simulink model "MARCH_v1"  (R2016a)
settings: Solver=FixedStepDiscrete  StartTime=0.0  StopTime=inf  FixedStep=0.001  RelTol=1e-3
PostLoadFcn:
  | build_location = fullfile(fileparts(which(bdroot)),'build');
  | 
  | set_param(0, 'CacheFolder', build_location);
  | set_param(0, 'CodeGenFolder', build_location);
InitFcn:
  | % Change dir to model location
  | cd(fileparts(which(bdroot)));
  | 
  | % Run init script
  | init_model;
StartFcn:
  | % Make sure we always move back to model folder
  | cd(fileparts(which(bdroot)));
StopFcn:
  | % Make sure we always move back to model folder
  | cd(fileparts(which(bdroot)));
libraries: xpcethercatlib x21
CloseFcn:
  | % Make sure we always move back to model folder
  | cd(fileparts(which(bdroot)));
  | 
  | set_param(0, 'CacheFolder', '');
  | set_param(0, 'CodeGenFolder', '');
PauseFcn:
  | % Make sure we always move back to model folder
  | cd(fileparts(which(bdroot)));
ContinueFcn:
  | % Make sure we always move back to model folder
  | cd(fileparts(which(bdroot)));
settings Model: xpc_rtwmakecfg_data=_xpcethercatlib_  Creator=Projectmarch  LastModifiedBy=Projectmarch
settings SolverCC: EnableConcurrentExecution=on  ConcurrentTasks=on  AutoInsertRateTranBlk=on
settings DataIOCC: LimitDataPoints=on  SaveFinalState=on  SaveFormat=StructureWithTime  InspectSignalLogs=on
settings OptimizationCC: BlockReduction=off  DefaultParameterBehavior=Inlined  OptimizeBlockIOStorage=off  BufferReuse=off  GlobalBufferReuse=off  ExpressionFolding=off  LocalBlockOutputs=off  StateBitsets=on  DataBitsets=on
settings DebuggingCC: AllowSymbolicDim=off
settings HardwareCC: ProdBitPerPointer=32  ProdLargestAtomicFloat=None  ProdWordSize=32  ProdLongLongMode=on  ProdHWDeviceType=Generic->32-bit x86 compatible
settings ModelReferenceCC: PropagateSignalLabelsOutOfModel=off
settings RTWCC: SystemTargetFile=slrt.tlc  TLCOptions=-p0  TemplateMakefile=slrt_default_tmf  Description=Simulink Real-Time  RTWVerbose=off  RTWCompilerOptimization=on
settings SimulinkRealTimeCC: xPCisModelTimeout=off  xPCModelTimeoutSecs=20

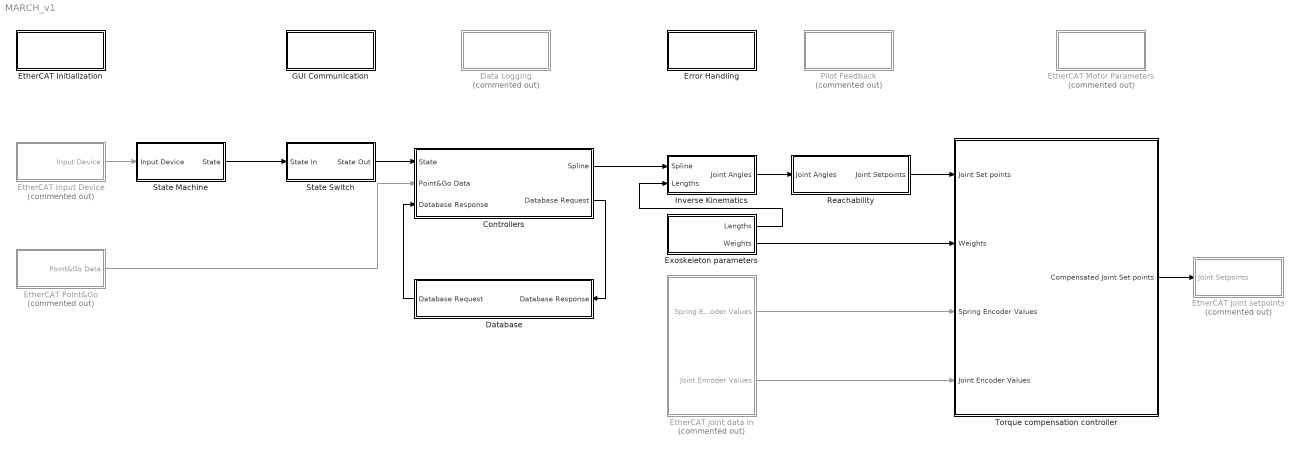
== system MARCH_v1 ==
  Controllers : Subsystem
  Data Logging : Subsystem  Commented=on
  Database : Subsystem
  Error Handling : Subsystem
  EtherCAT Initialization : Subsystem
  EtherCAT Input Device : Subsystem  Commented=on
  EtherCAT Motor Parameters : Subsystem  Commented=on
  EtherCAT Point&Go : Subsystem  Commented=on
  EtherCAT joint data in : Subsystem  Commented=on
  EtherCAT joint setpoints : Subsystem  Commented=on
  Exoskeleton parameters : Subsystem
  GUI Communication : Subsystem
  Inverse Kinematics : Subsystem
  Pilot Feedback : Subsystem  Commented=on
  Reachability : Subsystem
  State Machine : Subsystem
  State Switch : Subsystem
  Torque compensation controller : Subsystem
  wires:
  Torque compensation controller/1(Compensated Joint Set points) -> EtherCAT joint setpoints/1(Joint Setpoints)
  Reachability/1(Joint Setpoints) -> Torque compensation controller/1(Joint Set points)
  Inverse Kinematics/1(Joint Angles) -> Reachability/1(Joint Angles)
  State Switch/1(State Out) -> Controllers/1(State)
  Controllers/1(Spline) -> Inverse Kinematics/1(Spline)
  State Machine/1(State) -> State Switch/1(State In)
  Controllers/2(Database Request) -> Database/1(Database Response)
  Database/1(Database Request) -> Controllers/3(Database Response)
  EtherCAT joint data in/1(Spring Encoder Values) -> Torque compensation controller/3(Spring Encoder Values)
  EtherCAT joint data in/2(Joint Encoder Values) -> Torque compensation controller/4(Joint Encoder Values)
  Exoskeleton parameters/1(Lengths) -> Inverse Kinematics/2(Lengths)
  Exoskeleton parameters/2(Weights) -> Torque compensation controller/2(Weights)
  EtherCAT Input Device/1(Input Device) -> State Machine/1(Input Device)
  EtherCAT Point&Go/1(Point&Go Data) -> Controllers/2(Point&Go Data)

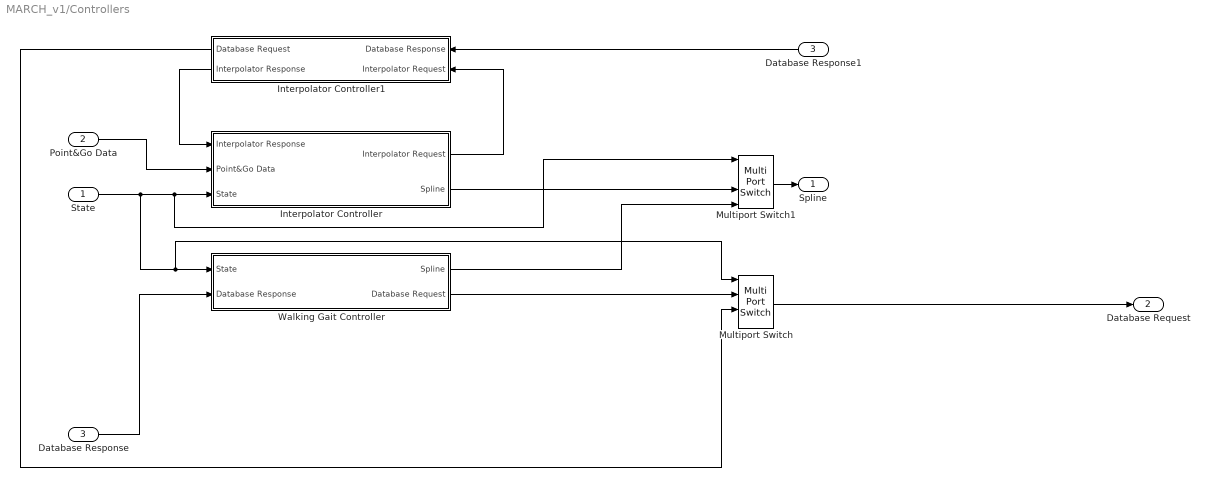
== system MARCH_v1/Controllers ==
  State : Inport
  Point&Go Data : Inport  Port=2
  Database Response : Inport  Port=3
  Database Response1 : InportShadow  Port=3
  Interpolator Controller : Subsystem
  Interpolator Controller1 : Subsystem
  Multiport Switch : MultiPortSwitch
  Multiport Switch1 : MultiPortSwitch
  Walking Gait Controller : Subsystem
  Spline : Outport
  Database Request : Outport  Port=2
  wires:
  State/1 -> Interpolator Controller/3(State), Multiport Switch1/1, Walking Gait Controller/1(State), Multiport Switch/1
  Database Response/1 -> Walking Gait Controller/2(Database Response)
  Walking Gait Controller/1(Spline) -> Multiport Switch1/4
  Interpolator Controller/1(Interpolator Request) -> Interpolator Controller1/2(Interpolator Request)
  Interpolator Controller1/2(Interpolator Response) -> Interpolator Controller/1(Interpolator Response)
  Database Response1/1 -> Interpolator Controller1/1(Database Response)
  Interpolator Controller1/1(Database Request) -> Multiport Switch/3
  Walking Gait Controller/2(Database Request) -> Multiport Switch/2
  Multiport Switch/1 -> Database Request/1
  Interpolator Controller/2(Spline) -> Multiport Switch1/3
  Multiport Switch1/1 -> Spline/1
  Point&Go Data/1 -> Interpolator Controller/2(Point&Go Data)

== system MARCH_v1/Data Logging ==

== system MARCH_v1/Database ==
  Database Response : Inport
  Database Request : Outport

== system MARCH_v1/Error Handling ==

== system MARCH_v1/EtherCAT Initialization ==
  "EtherCAT Init " : xpcethercatlib/EtherCAT Init   Priority=0  config_file=D:\Software\MATLAB\simulink-models\EtherCAT Config files\quad_slave_both_legs_v1.0.xml  device_id=0  pci_bus=0  pci_slot=0  dctuning=0  enaDebug=off  enaDC=on  errLink=off  masterDbg=off  stateChgDbg=off  baseClock=off  masterCfg=off  logFile='c:\dbglog.txt'  sample_time=0.001000

== system MARCH_v1/EtherCAT Input Device ==
  EtherCAT PDO Receive : xpcethercatlib/EtherCAT PDO Receive  Priority=2  sig_name=LHFE.Inputs.jointAngle  sig_offset=208  sig_type=uint32  type_size=32  sig_dim=1  device_id=0  sample_time=0.001000
  Input Device : Outport
  wires:
  EtherCAT PDO Receive/1 -> Input Device/1

== system MARCH_v1/EtherCAT Motor Parameters ==

== system MARCH_v1/EtherCAT Point&Go ==
  EtherCAT PDO Receive : xpcethercatlib/EtherCAT PDO Receive  Priority=2  sig_name=LHFE.Inputs.jointAngle  sig_offset=208  sig_type=uint32  type_size=32  sig_dim=1  device_id=0  sample_time=0.001000
  Point&Go Data : Outport
  wires:
  EtherCAT PDO Receive/1 -> Point&Go Data/1

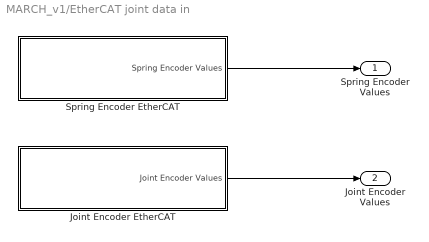
== system MARCH_v1/EtherCAT joint data in ==
  Joint Encoder EtherCAT : Subsystem
  Spring Encoder EtherCAT : Subsystem
  Spring Encoder Values : Outport
  Joint Encoder Values : Outport  Port=2
  wires:
  Spring Encoder EtherCAT/1(Spring Encoder Values) -> Spring Encoder Values/1
  Joint Encoder EtherCAT/1(Joint Encoder Values) -> Joint Encoder Values/1

== system MARCH_v1/EtherCAT joint setpoints ==
  Joint Setpoints : Inport
  EtherCAT Joint Communication : Subsystem
  wires:
  Joint Setpoints/1 -> EtherCAT Joint Communication/1(Joint Setpoints)

== system MARCH_v1/Exoskeleton parameters ==
  Lengths : Outport
  Weights : Outport  Port=2

== system MARCH_v1/GUI Communication ==

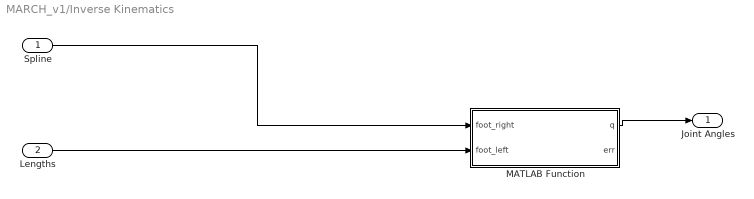
== system MARCH_v1/Inverse Kinematics ==
  Spline : Inport
  Lengths : Inport  Port=2
  MATLAB Function : MATLAB Function  TreatAsAtomicUnit=on
  Joint Angles : Outport
  wires:
  Spline/1 -> MATLAB Function/1(foot_right)
  MATLAB Function/1(q) -> Joint Angles/1
  Lengths/1 -> MATLAB Function/2(foot_left)

== system MARCH_v1/Pilot Feedback ==

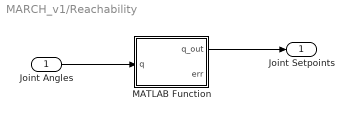
== system MARCH_v1/Reachability ==
  Joint Angles : Inport
  MATLAB Function : MATLAB Function  TreatAsAtomicUnit=on
  Joint Setpoints : Outport
  wires:
  Joint Angles/1 -> MATLAB Function/1(q)
  MATLAB Function/1(q_out) -> Joint Setpoints/1

== system MARCH_v1/State Machine ==
  Input Device : Inport
  Constant : Constant
  State : Outport
  wires:
  Constant/1 -> State/1

== system MARCH_v1/State Switch ==
  State In : Inport
  State Out : Outport
  wires:
  State In/1 -> State Out/1

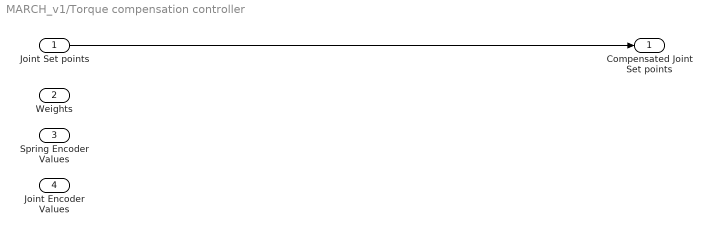
== system MARCH_v1/Torque compensation controller ==
  Joint Set points : Inport
  Weights : Inport  Port=2
  Spring Encoder Values : Inport  Port=3
  Joint Encoder Values : Inport  Port=4
  Compensated Joint Set points : Outport
  wires:
  Joint Set points/1 -> Compensated Joint Set points/1

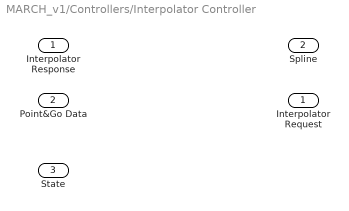
== system MARCH_v1/Controllers/Interpolator Controller ==
  Interpolator Response : Inport
  Point&Go Data : Inport  Port=2
  State : Inport  Port=3
  Interpolator Request : Outport
  Spline : Outport  Port=2

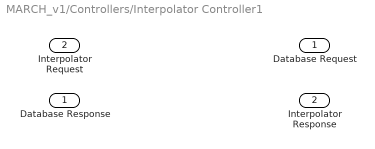
== system MARCH_v1/Controllers/Interpolator Controller1 ==
  Database Response : Inport
  Interpolator Request : Inport  Port=2
  Database Request : Outport
  Interpolator Response : Outport  Port=2

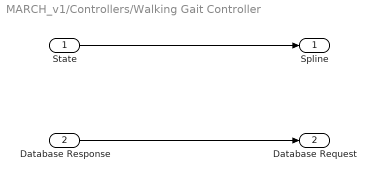
== system MARCH_v1/Controllers/Walking Gait Controller ==
  State : Inport
  Database Response : Inport  Port=2
  Spline : Outport
  Database Request : Outport  Port=2
  wires:
  State/1 -> Spline/1
  Database Response/1 -> Database Request/1

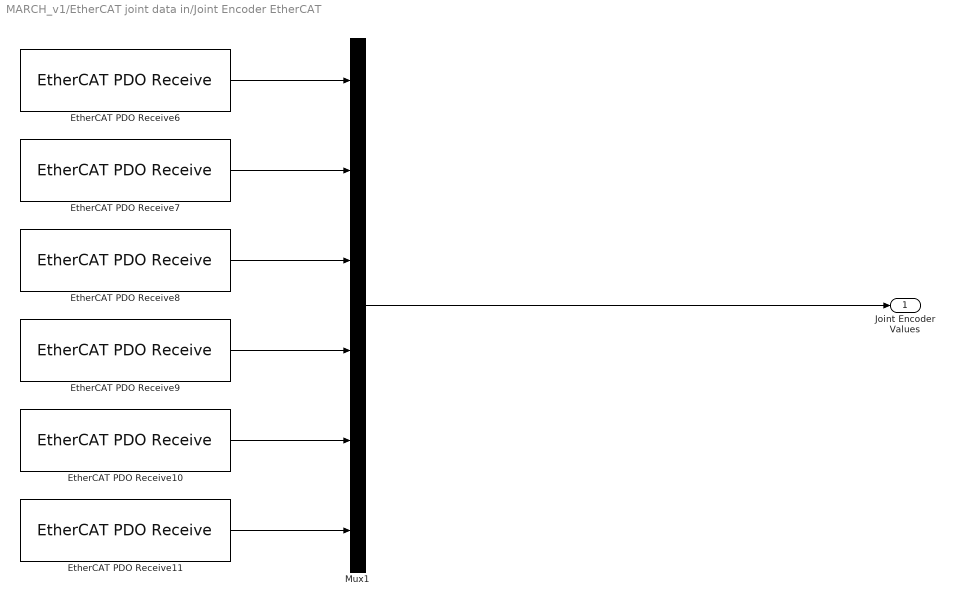
== system MARCH_v1/EtherCAT joint data in/Joint Encoder EtherCAT ==
  EtherCAT PDO Receive{6..11} (6 alike) : xpcethercatlib/EtherCAT PDO Receive  Priority=2  sig_name=Uninitialized Block  sig_offset=144  sig_type=uint8  type_size=8  sig_dim=1  device_id=0  sample_time=0.010000
  Mux1 : Mux  Inputs=6
  Joint Encoder Values : Outport
  wires:
  EtherCAT PDO Receive8/1 -> Mux1/3
  EtherCAT PDO Receive9/1 -> Mux1/4
  EtherCAT PDO Receive7/1 -> Mux1/2
  EtherCAT PDO Receive6/1 -> Mux1/1
  EtherCAT PDO Receive10/1 -> Mux1/5
  EtherCAT PDO Receive11/1 -> Mux1/6
  Mux1/1 -> Joint Encoder Values/1

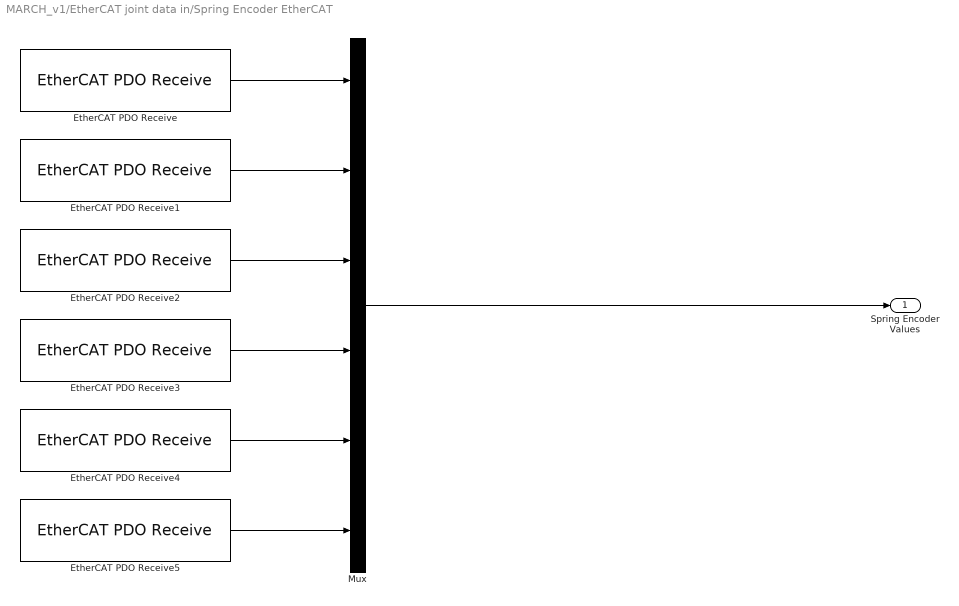
== system MARCH_v1/EtherCAT joint data in/Spring Encoder EtherCAT ==
  EtherCAT PDO Receive{,1..5} (6 alike) : xpcethercatlib/EtherCAT PDO Receive  Priority=2  sig_name=Uninitialized Block  sig_offset=144  sig_type=uint8  type_size=8  sig_dim=1  device_id=0  sample_time=0.010000
  Mux : Mux  Inputs=6
  Spring Encoder Values : Outport
  wires:
  EtherCAT PDO Receive2/1 -> Mux/3
  EtherCAT PDO Receive4/1 -> Mux/5
  Mux/1 -> Spring Encoder Values/1
  EtherCAT PDO Receive5/1 -> Mux/6
  EtherCAT PDO Receive1/1 -> Mux/2
  EtherCAT PDO Receive/1 -> Mux/1
  EtherCAT PDO Receive3/1 -> Mux/4

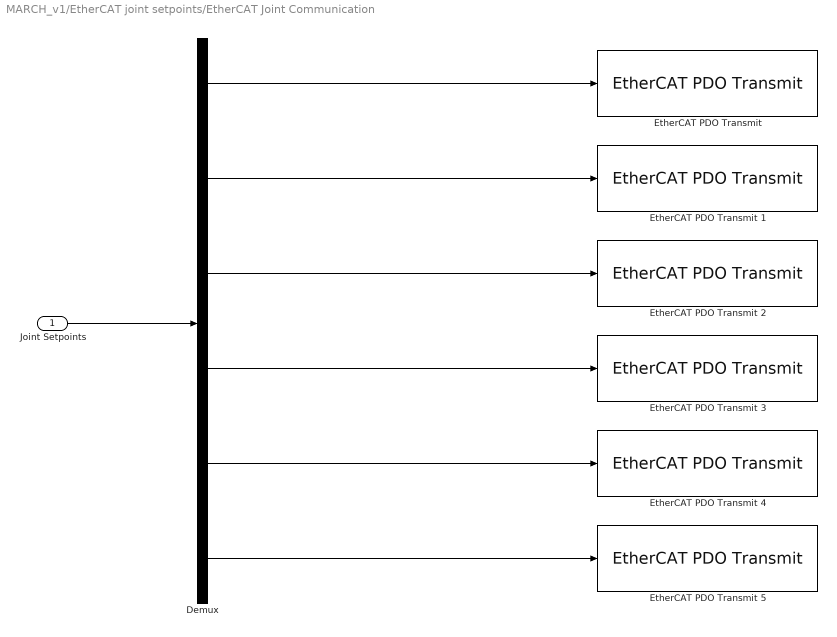
== system MARCH_v1/EtherCAT joint setpoints/EtherCAT Joint Communication ==
  Joint Setpoints : Inport
  Demux : Demux  Outputs=6
  "EtherCAT PDO Transmit " : xpcethercatlib/EtherCAT PDO Transmit   Priority=3  sig_name=LKFE.Outputs.jointSetpoint  sig_offset=496  sig_type=uint32  type_size=32  sig_dim=1  device_id=0  sample_time=0.001000
  EtherCAT PDO Transmit 1 : xpcethercatlib/EtherCAT PDO Transmit   Priority=3  sig_name=LHFE.Outputs.jointSetpoint  sig_offset=208  sig_type=uint32  type_size=32  sig_dim=1  device_id=0  sample_time=0.001000
  EtherCAT PDO Transmit 2 : xpcethercatlib/EtherCAT PDO Transmit   Priority=3  sig_name=Uninitialized Block  sig_offset=128  sig_type=uint8  type_size=8  sig_dim=1  device_id=0  sample_time=0.010000
  EtherCAT PDO Transmit 3 : xpcethercatlib/EtherCAT PDO Transmit   Priority=3  sig_name=Uninitialized Block  sig_offset=128  sig_type=uint8  type_size=32  sig_dim=1  device_id=0  sample_time=0.010000
  EtherCAT PDO Transmit 4 : xpcethercatlib/EtherCAT PDO Transmit   Priority=3  sig_name=RHFE.Outputs.jointSetpoint  sig_offset=12496  sig_type=uint32  type_size=32  sig_dim=1  device_id=0  sample_time=0.001
  EtherCAT PDO Transmit 5 : xpcethercatlib/EtherCAT PDO Transmit   Priority=3  sig_name=RKFE.Outputs.jointSetpoint  sig_offset=12784  sig_type=uint32  type_size=32  sig_dim=1  device_id=0  sample_time=0.001
  wires:
  Demux/5 -> EtherCAT PDO Transmit 4/1
  Demux/6 -> EtherCAT PDO Transmit 5/1
  Demux/4 -> EtherCAT PDO Transmit 3/1
  Demux/1 -> "EtherCAT PDO Transmit "/1
  Demux/3 -> EtherCAT PDO Transmit 2/1
  Demux/2 -> EtherCAT PDO Transmit 1/1
  Joint Setpoints/1 -> Demux/1

== matlab function MARCH_v1/Reachability/MATLAB Function ==
  data: q input; q_out output; err output
function [q_out, err] = fcn(q)

joint_limit_min = [-20 -109 -3 -23 -109 -3]/180*pi;
joint_limit_max = [23 21 121 20 21 121]/180*pi;

n = size(q,1);
%% Check if all joints are within limits

err = imag(q)~=0 | q<repmat(joint_limit_min,n,1) | q>repmat(joint_limit_max,n,1);
q_out = q;

== matlab function MARCH_v1/Inverse Kinematics/MATLAB Function ==
  data: foot_right input; q output; foot_left input; err output
function [q, err] = fcn(foot_right, foot_left)
%#codegen

inverse_kinematics(foot_right, foot_left);
q = 0;
err = 0;
